simulink model "IntelligentBinPicking"  (R2023a)
settings: Solver=FixedStepAuto  StartTime=0.0  StopTime=100  FixedStep=0.1  RelTol=1e-3
PreLoadFcn:
  | initializeParametersForBinPickingSimulationSL;
model workspace (MAT data in the model file):
  SL_ROS_VariableLengthArrays_MaxSizes : object (value not decoded)
undefined symbols (not defined in the file): binCenterPosition, Enable, enumCmd, getRBTFromUR, homePosition, IsAccValid, IsMoving, IsPosValid, isSingleDetection, IsValid, IsVelValid, JointAcc, JointCurrent, JointPos, JointTrajectory, JointVel, maxVisionObjects, Mode, motionPlannerCmdInitValue, motionPlannerResponseInitValue, NumObjects, NumPoints, objectDetectorResponseInitValue, Objects, ObjectTypesID, PickAllOrder, pickAllOrder, PickAndPlaceModes, PickSelectedObjectID, posTargetError, RequestID, Reset, RGBCameraTransform, robotCommandInitValue, robotFeedbackInitValue, ROSDeviceAddress, Status, targetEnv, TaskPlannerSampleTime, Time, TooltipTransform
libraries: robotlib x10, robotmaniplib x3, visionanalysis x2, robotcorelib x1, visiontextngfix x1, visionsinks x1
(part 2 of 2)

== system IntelligentBinPicking/Robot Command/Robot Command Subsystem/Actuator Commands/Hardware/Activate Vaccum Subsystem ==
  Enable : EnablePort
  Activate_Deactivate Vacuum : robotlib/Call Service  topicSource=Specify your own  service=/ur_hardware_interface/hand_back_control  serviceType=std_srvs/Trigger  connectionTimeout=5  keepPersistent=off  ShowErrorCodeOutput=on  legacyBusStruct=off
  Blank Message : robotlib/Blank Message  messageClass=Service Request  entityType=std_srvs/Trigger  messageType=std_srvs/TriggerRequest  SampleTime=inf  legacyBusStruct=off
  wires:
  Blank Message/1 -> Activate_Deactivate Vacuum/1

== matlab function IntelligentBinPicking/Object Detector/Object Detector/URSim_Hardware/MATLAB Function ==
  data: InputImage input; outputImage output
function outputImage = PreprocessImage(InputImage)
    networkInputSize = [416 416 3];
    originalInputSize = size(InputImage);

    % Input image resizing before passing it to the yolo detector. Its
    % recommended to keep this resize operation same as the resize
    % operation used while training the network
    resizeFactor = networkInputSize(1)/originalInputSize(2);
    offset = round((networkInputSize(1) - originalInputSize(1)*resizeFactor)/2);
    Tout =[ resizeFactor 0 0; 0 resizeFactor 0; 0 offset 1];
    tform = affine2d(Tout);
    outputImage = imwarp(InputImage,tform,...
        'OutputView',imref2d([networkInputSize(2) networkInputSize(1)]),...
        'SmoothEdges',true,...
        'FillValues',127);
end

== matlab function IntelligentBinPicking/Object Detector/Object Detector/URSim_Hardware/MATLAB Function1 ==
  data: bboxes input; bboxes output; rgbImage input
function bboxes = processBBoxes(bboxes,rgbImage)
    networkInputSize = [416 416 3];
    originalInputSize = size(rgbImage);
    resizeFactor = networkInputSize(1)/originalInputSize(2);

    offset = round((networkInputSize(1) - originalInputSize(1)*resizeFactor)/2);

    bboxes(:,2) = bboxes(:,2) - offset;
    topLeft = bboxes(:,1:2) - 1;
    topLeft = topLeft.*(size(rgbImage,2)./networkInputSize(2));
    bboxes = [topLeft + 1, bboxes(:,3:4).*(size(rgbImage,2)./networkInputSize(2))];
    
    % expand bounding boxes by few pixel if required
    bboxes(:,1:2) = bboxes(:,1:2)-5;
    bboxes(:,3:4) = bboxes(:,3:4)+5;
end

== matlab function IntelligentBinPicking/Object Detector/MATLAB Function ==
  data: objectDetectorResponseIn input Bus: BUS_object_detector_response; objectPose input; objectResponseOut output Bus: BUS_motion_planner_collision_object size=[maxVisionObjects 1]
function objectResponseOut = setObjectDetectedBus(objectDetectorResponseIn,objectPose)

objectResponseOut = objectDetectorResponseIn.Objects;
for i=1:size(objectPose,1)
    objectResponseOut(i).PickPos = objectPose(i, 1:3)';
    objectResponseOut(i).PickEulZYX = [objectPose(i, 4);0;0];
end

== stateflow chart IntelligentBinPicking/TaskPlanner/Chart ==
  state Setup
    entry:
    ii = 1;
    obsObjectCounter = 1;
    MotionPlannerCmd = motionPlannerCmdInitValue;
    RobotCommand = robotCommandInitValue;
    pickAllObjectIndex = uint32(1);
    objectToPickIndex  = uint32(0);
    objectPickedIndices = zeros(1,maxVisionObjects);
  state DeactivateVacuum
    entry:
    disp('Sending Deactivate Vacuum Command');
    RobotCommand.CommandToProcess = int32(enumCmd.deactivate_vacuum);
    RobotCommand.ProcessCommand = true;
    exit:
    RobotCommand.ProcessCommand = false;
  state SendToHome
    entry:
    disp('Sending robot to home position');
    RobotCommand.CommandToProcess = int32(enumCmd.send_to_home);
    RobotCommand.ProcessCommand = true;
    exit:
    RobotCommand.ProcessCommand = false;
  state DetectObjects
    state SendObjectDetectorRequest
      en: ObjectDetectorRequest;
      disp('Object Detection in Progress');
      %du: ObjectDetectorRequest;
    state ExtractObjectToPickSingleDetection
      en:
      motionCmdWithCollisionObjects = addCollisionObjectsInfo(ObjectDetectorResponse);
      generateDroppingPoses(ObjectDetectorResponse);
      [isObjectInScene, objectToPickPos, objectToPickEul, objectToPickIndex, pickAllObjectIndex] = getObjectToPick(UserCommand, ObjectDetectorResponse, pickAllObjectIndex);
    (junction 417) -> ExtractObjectToPickSingleDetection [order 1] : [isSingleDetection == true && UserCommand.Enable == true && ObjectDetectorResponse.Status == 1 && ...
        | ObjectDetectorResponse.NumObjects >= 1]
    (junction 417) -> SendObjectDetectorRequest [order 2]
    ExtractObjectToPickSingleDetection -> SendObjectDetectorRequest [order 3]
    SendObjectDetectorRequest -> ExtractObjectToPickSingleDetection [order 2] : [UserCommand.Enable == true && ObjectDetectorResponse.Status == 1 && ...
        | ObjectDetectorResponse.NumObjects >= 1]
    ExtractObjectToPickSingleDetection -> (junction 438) [order 2] : [isObjectInScene == true]
  state ObjectDetectorFailed
    entry:
    disp(" ");
    disp(" ");
    disp("No objects detected");
    disp(" ");
    disp("Stopping Simulation ");
    Stop();
  state StopSimulation
    entry:
    objectPickedIndices = zeros(1, maxVisionObjects);
    disp('No more objects to pick. Stopping simulation')
    Stop();
  state GoToPickingPose
    state GetPickingTrajectoryFromMotionPlanner
      entry:
      % Here based on object Pos and Eul get picking pose
      pickPos = objectToPickPos + [0.0; 0.0; 0.01];  % Bring the arm to 1cm above the pick position
      pickEul = objectToPickEul;
      %Create a motion planner task bus
      MotionPlannerCmd = createMotionTask(int32(objectToPickIndex), 'Pick', uint32(300), 0.2, RobotFeedback.JointPos, pickPos, [0 pi 0]');
      % Add obstacle objects
      MotionPlannerCmd.NumObstacleObjects = ObjectDetectorResponse.NumObjects - 1;
      ii= 1;
      obsObjectCounter = 1;
      for ii = 1:(ObjectDetectorResponse.NumObjects)
      if objectToPickIndex ~= ii
      MotionPlannerCmd.ObstacleObjects(obsObjectCounter) = ObjectDetectorResponse.Objects(ii);
      obsObjectCounter = obsObjectCounter + 1;
      end
      end
      % Send request to motion planner
      MotionPlannerRequest;
    state SendPickingTrajectoryToRobot
      entry:
      % Send trajectory to driver
      disp("Send traj to robot");
      RobotCommand.JointTrajectory = MotionPlannerResponse.JointTrajectory;
      RobotCommand.CommandToProcess = int32(enumCmd.precomputed_joint_trj);
      RobotCommand.ProcessCommand = true;
      posErr = Inf;
      orErr = Inf;
      success = false;
      during:
      RobotCommand.ProcessCommand = false;
      %  Check error and exit when tooltip reaches desired pose.
      T_task = eul2tform(pickEul');
      T_task(1:3,4) = pickPos;
      if targetEnv == TargetEnvs.Gazebo
      [posErr, orErr] = calcTaskSE3MaxError(T_task, RobotFeedback.TooltipTransform);
      if posErr < posTargetError
      success = true;
      end
      else
      success = ~RobotFeedback.IsMoving;
      end
      exit:
    GetPickingTrajectoryFromMotionPlanner -> (junction 14) : [MotionPlannerResponse.RequestID == MotionPlannerCmd.RequestID]
    (junction 14) -> SendPickingTrajectoryToRobot [order 1] : [MotionPlannerResponse.Status == 1 && ...
        | MotionPlannerResponse.IsPosValid == 1 && ...
        | MotionPlannerResponse.IsVelValid == 1 &&...
        |  MotionPlannerResponse.IsAccValid == 1]
  state ActivateVacuum
    entry:
    disp('Sending Activate Vacuum Command');
    RobotCommand.CommandToProcess = int32(enumCmd.activate_vacuum);
    RobotCommand.ProcessCommand = true;
    exit:
    RobotCommand.ProcessCommand = false;
  state MotionPlannerFailed
    en:
    RobotCommand.ProcessCommand = false;
    disp('Motion Planner failed');
  state GoToDroppingPose
    state RequestDroppingTrajectoryFromMotionPlanner
      entry:
      droppingPose = getDroppingPose(ObjectDetectorResponse,objectToPickIndex,droppingPoses, RobotFeedback.TooltipTransform);
      % Create motion planner task bus
      MotionPlannerCmd = createMotionTask(int32(objectToPickIndex), 'Place', uint32(300), 0.2, RobotFeedback.JointPos, droppingPose(1:3), droppingPose(4:6));
      % Add obstacle objects
      MotionPlannerCmd.NumObstacleObjects = ObjectDetectorResponse.NumObjects - 1;
      ii= 1;
      obsObjectCounter = 1;
      for ii = 1:(ObjectDetectorResponse.NumObjects)
      if objectToPickIndex ~= ii
      MotionPlannerCmd.ObstacleObjects(obsObjectCounter) = ObjectDetectorResponse.Objects(ii);
      obsObjectCounter = obsObjectCounter + 1;
      end
      end
      % Send request to motion planner
      MotionPlannerRequest;
    state SendDroppingTrajectoryToRobot
      entry:
      % Send trajectory to driver
      RobotCommand.JointTrajectory = MotionPlannerResponse.JointTrajectory;
      RobotCommand.CommandToProcess = int32(enumCmd.precomputed_joint_trj);
      RobotCommand.ProcessCommand = true;
      posErr = Inf;
      orErr = Inf;
      success = false;
      during:
      RobotCommand.ProcessCommand = false;
      %  Check error and exit when tooltip reaches desired pose.
      T_task = eul2tform(droppingPose(4:6)');
      T_task(1:3,4) = droppingPose(1:3);
      if targetEnv == TargetEnvs.Gazebo
      [posErr, orErr] = calcTaskSE3MaxError(T_task, RobotFeedback.TooltipTransform);
      if posErr < posTargetError
      success = true;
      end
      else
      success = ~RobotFeedback.IsMoving;
      end
      exit:
    RequestDroppingTrajectoryFromMotionPlanner -> (junction 128) : [MotionPlannerResponse.RequestID == MotionPlannerCmd.RequestID]
    (junction 128) -> SendDroppingTrajectoryToRobot [order 1] : [MotionPlannerResponse.Status == 1 && ...
        | MotionPlannerResponse.IsPosValid == 1 && ...
        | MotionPlannerResponse.IsVelValid == 1 && ...
        | MotionPlannerResponse.IsAccValid == 1]
  state Stop [function]
  SendPickingTrajectoryToRobot -> ActivateVacuum : [success == true]
  SendToHome -> (junction 417)
  ActivateVacuum -> RequestDroppingTrajectoryFromMotionPlanner : {pause(0.5)}
  ExtractObjectToPickSingleDetection -> StopSimulation [order 1] : [objectToPickIndex == uint32(-1)]
  (junction 438) -> GetPickingTrajectoryFromMotionPlanner : {pause(1)}
  (junction 259) -> Setup
  (default) -> Setup
  (junction 258) -> (junction 259)
  Setup -> (junction 498) : [UserCommand.Enable == true && RobotFeedback.IsValid]
  (junction 498) -> (junction 500) [order 2] : [nnz(objectPickedIndices) == 0]
  (junction 498) -> DeactivateVacuum [order 1] : [nnz(objectPickedIndices) > 0]
  (junction 500) -> SendToHome
  (junction 253) -> DeactivateVacuum
  (junction 485) -> (junction 253)
  DeactivateVacuum -> SendToHome : {pause(1)}
  SendDroppingTrajectoryToRobot -> (junction 256) : [success == true]
  SendObjectDetectorRequest -> ObjectDetectorFailed [order 1] : [ObjectDetectorResponse.Status == -1]
  MotionPlannerFailed -> (junction 258)
  (junction 256) -> (junction 485)
  (junction 128) -> MotionPlannerFailed [order 2]
  (junction 14) -> MotionPlannerFailed [order 2]
  data: requestIDIn function_input; typeIn function_input; maxIterationsIn function_input; sampleTimeIn function_input; q0In function_input; targetPosIn function_input; targetEulIn function_input; motionPlannerCmdOut function_output; T_aIn function_input double size=[4 4]; T_bIn function_input double size=[4 4]; posErrOut function_output double size=1; orErrOut function_output double size=1; objectDetectorResponse function_input; droppingPoseOut function_output double size=[6 1]; objectDetectorResponseIn function_input Bus: BUS_object_detector_response size=1; objectToPickIndexIn function_input; droppingPosesIn function_input size=[6, maxVisionObjects]; tooltipTransformIn function_input; detectorResponse function_input; motionCmd function_output; userCommandIn function_input Bus: BUS_user_command size=1; objectDetectorResponseIn function_input Bus: BUS_object_detector_response size=1; isObjectInSceneOut function_output; objectToPickPosOut function_output double size=[3 1]; objectToPickEulOut function_output double size=[3 1]; objectToPickIndexOut function_output uint32 size=1; pickAllObjectIndexOut function_output uint32 size=1; pickAllObjectIndexIn function_input uint32 size=1; RobotCommand output Bus: BUS_robot_command size=1; UserCommand input Bus: BUS_user_command size=1; ObjectDetectorResponse input Bus: BUS_object_detector_response size=1; motionPlannerCmdInitValue parameter size=1; MotionPlannerResponse input Bus: BUS_motion_planner_response size=1; MotionPlannerCmd output Bus: BUS_motion_planner_cmd size=1; isObjectInScene local boolean size=1 =false; objectToPickEul local; objectToPickPos local; ii local uint32 size=1; obsObjectCounter local uint32 size=1; RobotFeedback input Bus: BUS_robot_feedback size=1; T_task local double size=[4, 4]; orErr local double size=1; posErr local double size=1; posTargetError parameter double size=1; droppingPoses local double size=[6, maxVisionObjects] =zeros(6, maxVisionObjects); pickEul local double size=[3 1]; pickPos local double size=[3 1]; pickAllObjectIndex local uint32 size=1; objectToPickIndex local uint32 size=1; droppingPose local double size=[6 1]; robotCommandInitValue parameter size=1; isSingleDetection parameter; binCenterPosition parameter; objectPickedIndices local double size=[1 maxVisionObjects] =zeros(1, maxVisionObjects); targetEnv parameter; motionCmdWithCollisionObjects local Bus: BUS_motion_planner_cmd size=1; success local; maxVisionObjects parameter double size=1
  events: MotionPlannerRequest output FUNCTION_CALL_EVENT; ObjectDetectorRequest output FUNCTION_CALL_EVENT
  function motionPlannerCmdOut = createMotionTask(requestIDIn, typeIn, maxIterationsIn, sampleTimeIn, q0In, targetPosIn, targetEulIn):
    | function motionPlannerCmdOut = createMotionTask(requestIDIn, typeIn, maxIterationsIn, sampleTimeIn, q0In, targetPosIn, targetEulIn)
    | 
    | % In this one I didn't expose the max velocity because the planner doesn't
    | % consider the acceleration limits directly. We use a conservative Lin and
    | % Ang limits to control acceleration.
    | 
    | % q0In = [q0In; 0; 0; 0; 0; 0; 0;];
    | 
    | % Initialize bus
    | motionPlannerCmdOut = motionCmdWithCollisionObjects;
    | 
    | % Configure motion planner tasks
    | motionPlannerCmdOut.RequestID = requestIDIn;
    | motionPlannerCmdOut.NumTasks = uint32(4);
    | motionPlannerCmdOut.MaxIterations = maxIterationsIn;
    | motionPlannerCmdOut.SampleTime = sampleTimeIn;
    | motionPlannerCmdOut.InitialPositions = q0In;
    | % Task 1: End effector pose
    | motionPlannerCmdOut.Tasks(1).Name(1:length(uint8('TooltipTaskSE3'))) = uint8('TooltipTaskSE3');
    | motionPlannerCmdOut.Tasks(1).Type(1:length(typeIn))  = uint8(typeIn);
    | motionPlannerCmdOut.Tasks(1).FrameName(1:length(uint8('Bellow')))  = uint8('Bellow');
    | motionPlannerCmdOut.Tasks(1).p = targetPosIn;
    | motionPlannerCmdOut.Tasks(1).eulZYX = targetEulIn;
    | motionPlannerCmdOut.Tasks(1).MaxLinVel = 0.10;  % 0.072 0.1 0.15
    | motionPlannerCmdOut.Tasks(1).MaxAngVel = 0.4;    % 0.4
    | motionPlannerCmdOut.Tasks(1).Weight = 1.0;
    | motionPlannerCmdOut.Tasks(1).MaxLinError = 0.01;        % 0.01
    | motionPlannerCmdOut.Tasks(1).MaxAngError = deg2rad(2);  % 2
  function [posErrOut,orErrOut] = calcTaskSE3MaxError(T_aIn, T_bIn):
    | function [posErrOut,orErrOut] = calcTaskSE3MaxError(T_aIn, T_bIn)
    |  
    | % Position error is max of coordinate
    | posErrOut = max(abs(T_aIn(1:3,4) - T_bIn(1:3,4)));
    | 
    | % Orientation error with quaternions. Also using max for error
    | q_a = tform2quat(T_aIn);
    | q_b = tform2quat(T_bIn);
    | 
    | % skew
    | S_a = [      0, -q_a(4),  q_a(3); 
    |         q_a(4),       0, -q_a(2); 
    |        -q_a(3),  q_a(2),       0];
    |     
    | or_error = q_b(1)*q_a(2:4)'-q_a(1)*q_b(2:4)'- S_a*q_b(2:4)';    % q = [w x y z]
    | 
    | orErrOut = max(abs(or_error));
  function generateDroppingPoses(objectDetectorResponse):
    | function generateDroppingPoses(objectDetectorResponse)
    |  
    | %% Define dropping poses
    | 
    | 
    | %For single detection workflow, the dropping poses will get defined once
    | %and then used in the getDroppingPoses method.
    | 
    | %For multiple detections, ensure that the dropping poses get generated only
    | %once. Check the presence of non-zero value in objectPickedIndices to
    | %detect subsequent detections.
    | 
    | %In this implementation, the user defined drop POSITION doesn't change based
    | %on the pose of the object before picking. However, the orientation of the object
    | %may change during the course of picking other objects and that is taken
    | %into account in the getDroppingPose method.
    | 
    | %Generate dropping pose only once
    | if isempty(find(objectPickedIndices,1))
    |     numOfParts = objectDetectorResponse.NumObjects;
    |     droppingPoses = zeros(6, maxVisionObjects);
    |     for i=1:numOfParts
    |         if i>numOfParts-1
    |             droppingPoses(:, i) = [0.01 0.59 -0.018 0 pi 0]';
    |         else
    |             droppingPoses(:, i) = [0.01+(double(i)-1)*0.07 0.75 -0.018 0 pi 0]';
    |         end
    |     end
    | end
  function droppingPoseOut = getDroppingPose(objectDetectorResponseIn,objectToPickIndexIn,droppingPosesIn, tooltipTransformIn):
    | function droppingPoseOut = getDroppingPose(objectDetectorResponseIn,objectToPickIndexIn,droppingPosesIn, tooltipTransformIn)
    | 
    | % Use the number of objects already picked to determine the dropping pose
    | % for the current object
    | droppingPoseIdxToUse = numel(find(objectPickedIndices));
    | 
    | droppingPoseOut = droppingPosesIn(:,droppingPoseIdxToUse);
    | eulAtApproach = tform2eul(tooltipTransformIn);
    | 
    | %Take into account the orientation of the object in the bin
    | droppingPoseOut(4) = abs(eulAtApproach(1)) - deg2rad(objectDetectorResponseIn.Objects(objectToPickIndexIn).PickEulZYX(1));
  function motionCmd = addCollisionObjectsInfo(detectorResponse):
    | function motionCmd = addCollisionObjectsInfo(detectorResponse)
    | 
    | motionCmd = motionPlannerCmdInitValue;
    | 
    | numObjectsToPick = detectorResponse.NumObjects;
    | motionCmd.NumObstacleObjects = numObjectsToPick;
    | 
    | for ii = 1:numObjectsToPick
    |    motionCmd.ObstacleObjects(ii) = detectorResponse.Objects(ii);
    | end
    | 
    | 
    | end
  function [isObjectInSceneOut, objectToPickPosOut, objectToPickEulOut, objectToPickIndexOut, pickAllObjectIndexOut]=  getObjectToPick(userCommandIn,objectDetectorResponseIn, pickAllObjectIndexIn):
    | function [isObjectInSceneOut, objectToPickPosOut, objectToPickEulOut, objectToPickIndexOut, pickAllObjectIndexOut]=  getObjectToPick(userCommandIn,objectDetectorResponseIn, pickAllObjectIndexIn)
    |  
    | isObjectInSceneOut = false;
    | objectToPickPosOut = zeros(3,1);
    | objectToPickEulOut = zeros(3,1);
    | objectToPickIndexOut = uint32(0);
    | pickAllObjectIndexOut = pickAllObjectIndexIn;
    | 
    | %If a single detection is being done, then we need to keep track of which
    | %objects were picked, objectPickedIndices. On the othe rhand, when doing a
    | %detection after each pick and place operation, we just need to pick up the
    | %object closest to the center of the bin.
    | if isSingleDetection
    |     % List of parts poses that are still in the bin
    |     partsToPickGT = zeros(objectDetectorResponseIn.NumObjects - nnz(objectPickedIndices), 6);
    |     if ~isempty(partsToPickGT)
    |         partsToPickGTIdx = 1;
    |         partsToPickDetectedIdx = zeros(1,10);
    |         for ii = 1:objectDetectorResponseIn.NumObjects
    |             %If the part has been picked, don't use its pose
    |             if ~any(objectPickedIndices == ii)
    |                 partsToPickGT(partsToPickGTIdx, 1:3) = objectDetectorResponseIn.Objects(ii).PickPos;
    |                 partsToPickGT(partsToPickGTIdx, 4) = objectDetectorResponseIn.Objects(ii).PickEulZYX(1);
    |                 partsToPickDetectedIdx(partsToPickGTIdx) = ii;
    |                 partsToPickGTIdx = partsToPickGTIdx + 1;
    |             end
    |         end
    | 
    |         [refPose,partIDToPick] = exampleHelperSelectPartForMEXPlanner(partsToPickGT,binCenterPosition);
    |         
    |         if ~isempty(refPose)
    |             isObjectInSceneOut = true;
    |             objectToPickPosOut = refPose';
    |             objectToPickEulOut = [0 pi 0]';
    |             objectToPickIndexOut = uint32(partsToPickDetectedIdx(partIDToPick));
    |             if pickAllObjectIndexIn < length(userCommandIn.PickAllOrder)
    |                 pickAllObjectIndexOut = pickAllObjectIndexIn + 1;
    |             else
    |                 pickAllObjectIndexOut = uint32(1);
    |             end
    | 
    |             if size(partsToPickGT, 1) == objectDetectorResponseIn.NumObjects
    |                 objectPickedIndices(1) = objectToPickIndexOut;
    |             else
    |                 objectPickedIndices(find(objectPickedIndices, 1, 'Last') + 1) = objectToPickIndexOut;
    |             end
    |         end
    |     else
    |         objectToPickIndexOut = uint32(-1);
    |     end
    | 
    | else
    |     partsToPickGT = zeros(objectDetectorResponseIn.NumObjects, 6);
    |     if ~isempty(partsToPickGT)
    |         for ii = 1:objectDetectorResponseIn.NumObjects
    |             partsToPickGT(ii, 1:3) = objectDetectorResponseIn.Objects(ii).PickPos;
    |             partsToPickGT(ii, 4) = objectDetectorResponseIn.Objects(ii).PickEulZYX(1);
    |         end
    | 
    |         [refPose,partIDToPick] = exampleHelperSelectPartForMEXPlanner(partsToPickGT,binCenterPosition);
    | 
    |         if ~isempty(refPose)
    |             isObjectInSceneOut = true;
    |             objectToPickPosOut = refPose';
    |             objectToPickEulOut = [0 pi 0]';
    |             objectToPickIndexOut = uint32(partIDToPick);
    |             if pickAllObjectIndexIn < length(userCommandIn.PickAllOrder)
    |                 pickAllObjectIndexOut = pickAllObjectIndexIn + 1;
    |             else
    |                 pickAllObjectIndexOut = uint32(1);
    |             end
    | 
    |             if isempty(find(objectPickedIndices,1))
    |                 objectPickedIndices(1) = partIDToPick;
    |             else
    |                 objectPickedIndices(find(objectPickedIndices, 1, 'Last') + 1) = partIDToPick;
    |             end
    |         end
    |     else
    |         objectToPickIndexOut = uint32(-1);
    |     end
    | end
